simulink model "Velocity"  (R2023b)
settings: Solver=VariableStepAuto  StartTime=0.0  StopTime=10.0  RelTol=1e-3
undefined symbols (not defined in the file): g
libraries: simulink x3, eeGeneralControl x1
settings Model: Creator=Saif Mohamed  LastModifiedBy=saifg

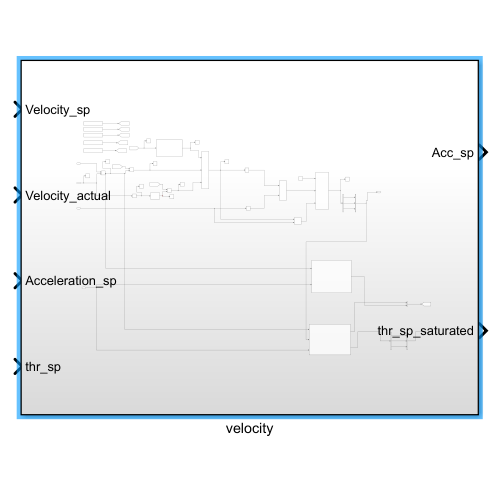
[thumbnail: Simulink's stored preview of the top-level diagram]
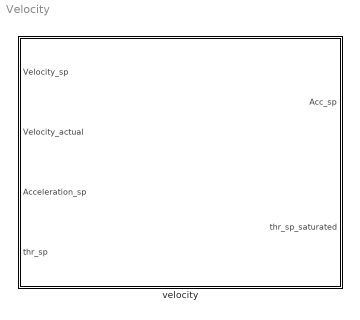
== system Velocity ==
  velocity : Subsystem

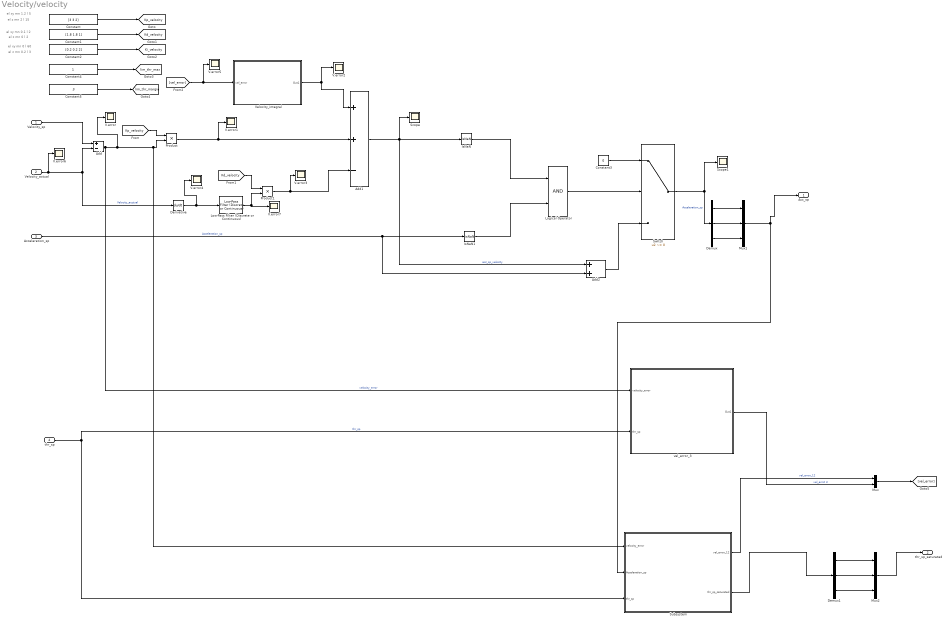
== system Velocity/velocity ==
  note: el z mn 0.2 l 3
  note: el xy mn 0 l 60
  note: el xy mn 0.1 l 2
  note: el z mn 0 l 2
  note: el xy mn 1.2 l 5
  note: el z mn 2 l 15
  Velocity_sp : Inport
  Velocity_actual : Inport  Port=2
  Acceleration_sp : Inport  Port=3
  thr_sp : Inport  Port=4
  Add : Sum  Inputs=+-
  Add1 : Sum  Inputs=++-
  Add2 : Sum
  Constant : Constant  Value=[3 3 2]
  Constant1 : Constant  Value=[1.8 1.8 1]
  Constant2 : Constant  Value=[0.2 0.2 2]
  Constant3 : Constant  Value=0
  Constant4 : Constant
  Constant5 : Constant  Value=.3
  Demux : Demux  Outputs=3
  Demux1 : Demux  Outputs=3
  Derivative : Derivative
  IsNaN : RelationalOperator  Operator=isNaN  OutDataTypeStr=boolean  RndMeth=Simplest  InputSameDT=off
  IsNaN1 : RelationalOperator  Operator=isNaN  OutDataTypeStr=boolean  RndMeth=Simplest  InputSameDT=off
  Logical Operator : Logic  AllPortsSameDT=off  OutDataTypeStr=boolean
  Low-Pass Filter (Discrete or Continuous) : eeGeneralControl/Low-Pass Filter (Discrete or Continuous)  K=1  T=1  B=inf  A=-inf  init_option=Inherited from block input  x0=0  Ts=-1
  Mux : Mux  Inputs=2
  Mux1 : Mux  Inputs=3
  Mux2 : Mux  Inputs=3
  Product : Product
  Product1 : Product
  Scope : Scope
  Scope1 : Scope
  Subsystem : Subsystem
  Switch : Switch  Criteria=u2 ~= 0  SaturateOnIntegerOverflow=off  InputSameDT=off
  V.error{,1..7} (8 alike) : Scope
  Velocity_integral : Subsystem
  vel_error_3 : Subsystem
  Acc_sp : Outport
  thr_sp_saturated : Outport  Port=2
  tag scope: Kd_velocity=global, Ki_velocity=global, Kp_velocity=global, lim_thr_margin=global, lim_thr_max=global
  wires:
  Velocity_sp/1 -> Add/1
  Velocity_actual/1 -> V.error6/1, Derivative/1, Add/2  "Velocity_acctual"
  Add/1 -> vel_error_3/1(velocity_error), V.error/1, Subsystem/1(velocity_error), Product/2  "velocity_error"
  Constant/1 -> [Kp_velocity]
  [Kp_velocity] -> Product/1
  Derivative/1 -> V.error4/1, Low-Pass Filter (Discrete or Continuous)/1
  Constant1/1 -> [Kd_velocity]
  Low-Pass Filter (Discrete or Continuous)/1 -> V.error7/1, Product1/2
  [Kd_velocity] -> Product1/1
  Constant2/1 -> [Ki_velocity]
  Add1/1 -> Scope/1, IsNaN/1, Add2/1  "acc_sp_velocity"
  Acceleration_sp/1 -> Add2/2, IsNaN1/1  "Acceleration_sp"
  IsNaN1/1 -> Logical Operator/2
  IsNaN/1 -> Logical Operator/1
  Logical Operator/1 -> Switch/2
  Add2/1 -> Switch/3
  Constant3/1 -> Switch/1
  Switch/1 -> Scope1/1, Demux/1  "Acceleration_sp"
  Constant4/1 -> [lim_thr_max]
  thr_sp/1 -> Subsystem/3(thr_sp), vel_error_3/2(thr_sp)  "thr_sp"
  vel_error_3/1(Out1) -> Mux/2  "vel_errot 3"
  Constant5/1 -> [lim_thr_margin]
  Subsystem/1(vel_error_12) -> Mux/1  "vel_error_12"
  Mux/1 -> [vel_error]
  Demux/3 -> Mux1/3
  Demux/2 -> Mux1/2
  Demux/1 -> Mux1/1
  Demux1/1 -> Mux2/1
  Demux1/2 -> Mux2/2
  Subsystem/2(thr_sp_satureted) -> Demux1/1
  Mux2/1 -> thr_sp_saturated/1
  Demux1/3 -> Mux2/3
  Product/1 -> Add1/2, V.error1/1
  Velocity_integral/1(Out1) -> Add1/1, V.error2/1
  Product1/1 -> Add1/3, V.error3/1
  Mux1/1 -> Subsystem/2(Acceleration_sp), Acc_sp/1
  [vel_error] -> Velocity_integral/1(vel_error), V.error5/1

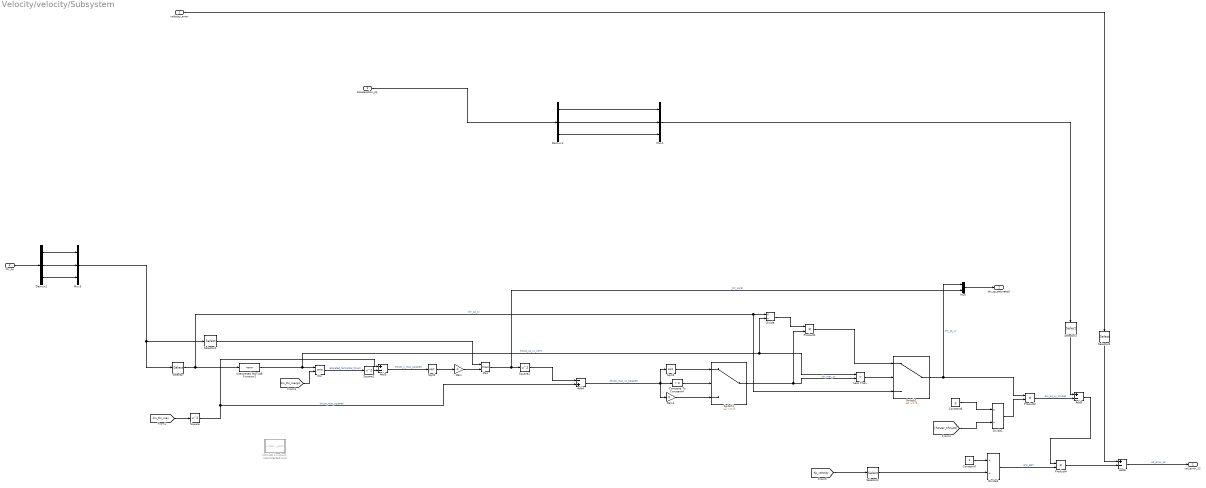
== system Velocity/velocity/Subsystem ==
  velocity_error : Inport
  Acceleration_sp : Inport  Port=2
  thr_sp : Inport  Port=3
  Add3 : Sum  Inputs=+-
  Add4 : Sum  Inputs=-+
  Add5 : Sum  Inputs=+-
  Add6 : Sum  Inputs=+-
  Compare To Constant4 : simulink/Logic and Bit Operations/Compare To Constant  relop=>  const=0  OutDataTypeStr=boolean
  Constant6 : Constant  Value=g
  Constant7 : Constant  Value=2
  Demux1 : Demux  Outputs=3
  Demux2 : Demux  Outputs=3
  Divide : Product  Inputs=*/
  Divide1 : Product  Inputs=*/
  Divide2 : Product  Inputs=*/
  Gain : Gain  Gain=-1
  Gain1 : Gain  Gain=0
  Interpreted MATLAB Function1 : MATLABFcn  MATLABFcn=norm
  Less Than : RelationalOperator  Operator=>  OutDataTypeStr=boolean  RndMeth=Simplest  InputSameDT=off
  MATLAB Function1 : MATLAB Function  Commented=on  TreatAsAtomicUnit=on
  Max : MinMax  Function=max  Inputs=2
  Min : MinMax  Inputs=2
  Mux : Mux  Inputs=2
  Mux1 : Mux  Inputs=3
  Mux3 : Mux  Inputs=3
  Product2 : Product
  Product3 : Product
  Product4 : Product
  Selector : Selector  InputPortWidth=3  IndexOptions=Index vector (dialog)  Indices=[1 2]  OutputSizes=1
  Selector1 : Selector  InputPortWidth=3  IndexOptions=Index vector (dialog)  Indices=[3]  OutputSizes=1
  Selector2 : Selector  InputPortWidth=3  IndexOptions=Index vector (dialog)  Indices=[1]  OutputSizes=1
  Selector3 : Selector  InputPortWidth=3  IndexOptions=Index vector (dialog)  Indices=[1 2]  OutputSizes=1
  Selector4 : Selector  InputPortWidth=3  IndexOptions=Index vector (dialog)  Indices=[1 2]  OutputSizes=1
  Sqrt1 : Sqrt
  Sqrt3 : Sqrt
  Square : Math  Operator=square
  Square1 : Math  Operator=square
  Square2 : Math  Operator=square
  Switch1 : Switch  Criteria=u2 ~= 0  Threshold=~0  SaturateOnIntegerOverflow=off  InputSameDT=off
  Switch2 : Switch  Criteria=u2 ~= 0  Threshold=~0  SaturateOnIntegerOverflow=off  InputSameDT=off
  vel_error_12 : Outport
  thr_sp_satureted : Outport  Port=2
  wires:
  Square/1 -> Add4/2, Add3/1  "thrust_max_squared"
  Divide2/1 -> Product4/2  "arw_gain"
  Selector/1 -> Interpreted MATLAB Function1/1, Switch2/3, Divide/1  "thr_sp_xy"
  Add5/1 -> Product4/1
  Max/1 -> Square2/1, Mux/2  "_thr_sp(3)"
  Product4/1 -> Add6/2
  Divide/1 -> Product2/1
  Compare To Constant4/1 -> Switch1/2
  Sqrt3/1 -> Switch1/1
  Selector4/1 -> Add6/1
  Switch2/1 -> Mux/1, Product3/1  "thr_sp_xy"
  Interpreted MATLAB Function1/1 -> Divide/2, Less Than/1, Min/1  "thrust_sp_xy_norm"
  Add4/1 -> Gain1/1, Sqrt3/1, Compare To Constant4/1  "thrust_max_xy_squared"
  Selector1/1 -> Max/1
  Sqrt1/1 -> Gain/1
  Selector2/1 -> Divide2/2
  Switch1/1 -> Product2/2, Less Than/2  "thr_max_xy"
  [lim_thr_max] -> Square/1
  [hover_thrust] -> Divide1/2
  Add3/1 -> Sqrt1/1  "thrust_z_max_squared"
  Selector3/1 -> Add5/1
  Gain/1 -> Max/2
  [lim_thr_margin] -> Min/2
  Product2/1 -> Switch2/1
  Product3/1 -> Add5/2  "acc_sp_xy_limited"
  [Kp_velocity] -> Selector2/1
  Square2/1 -> Add4/1
  Less Than/1 -> Switch2/2
  Constant7/1 -> Divide2/1
  Min/1 -> Square1/1  "allocated_horizontal_thrust"
  Divide1/1 -> Product3/2
  Add6/1 -> vel_error_12/1  "vel_error_12"
  velocity_error/1 -> Selector4/1
  Square1/1 -> Add3/2
  Constant6/1 -> Divide1/1
  Gain1/1 -> Switch1/3
  Mux/1 -> thr_sp_satureted/1
  Demux2/1 -> Mux3/1
  Demux2/2 -> Mux3/2
  Mux3/1 -> Selector/1, Selector1/1
  thr_sp/1 -> Demux2/1
  Demux2/3 -> Mux3/3
  Mux1/1 -> Selector3/1
  Acceleration_sp/1 -> Demux1/1
  Demux1/3 -> Mux1/3
  Demux1/2 -> Mux1/2
  Demux1/1 -> Mux1/1

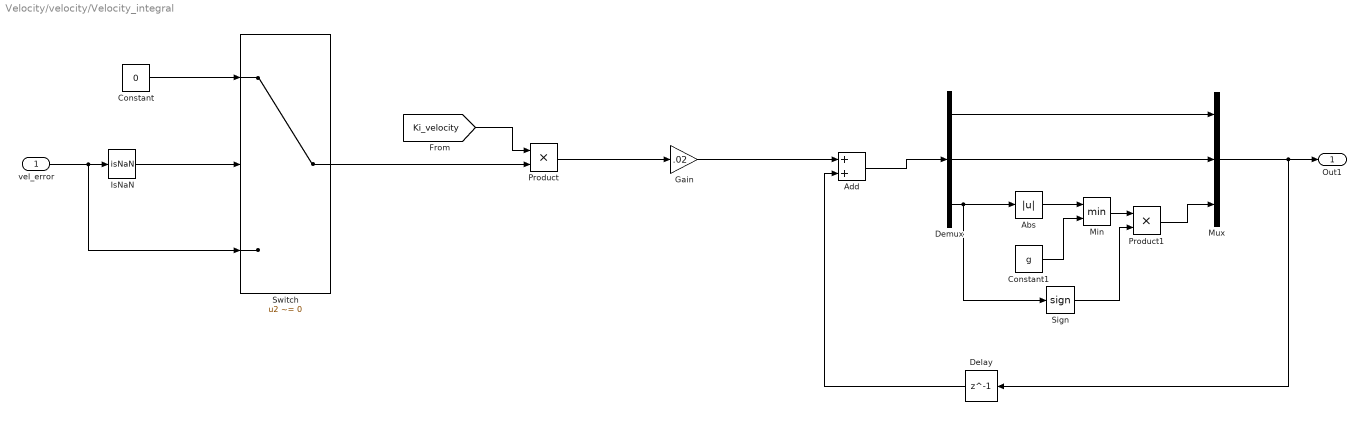
== system Velocity/velocity/Velocity_integral ==
  vel_error : Inport
  Abs : Abs  SaturateOnIntegerOverflow=off
  Add : Sum
  Constant : Constant  Value=0
  Constant1 : Constant  Value=g
  Delay : Delay  DelayLength=1
  Demux : Demux  Outputs=3
  Gain : Gain  Gain=.02
  IsNaN : RelationalOperator  Operator=isNaN  OutDataTypeStr=boolean  RndMeth=Simplest  InputSameDT=off
  Min : MinMax  Inputs=2
  Mux : Mux  Inputs=3
  Product : Product
  Product1 : Product
  Sign : Signum
  Switch : Switch  Criteria=u2 ~= 0  SaturateOnIntegerOverflow=off  InputSameDT=off
  Out1 : Outport
  wires:
  vel_error/1 -> Switch/3, IsNaN/1
  IsNaN/1 -> Switch/2
  Constant/1 -> Switch/1
  [Ki_velocity] -> Product/1
  Switch/1 -> Product/2
  Delay/1 -> Add/2
  Min/1 -> Product1/1
  Constant1/1 -> Min/2
  Product1/1 -> Mux/3
  Abs/1 -> Min/1
  Gain/1 -> Add/1
  Demux/3 -> Sign/1, Abs/1
  Sign/1 -> Product1/2
  Add/1 -> Demux/1
  Product/1 -> Gain/1
  Demux/2 -> Mux/2
  Demux/1 -> Mux/1
  Mux/1 -> Out1/1, Delay/1

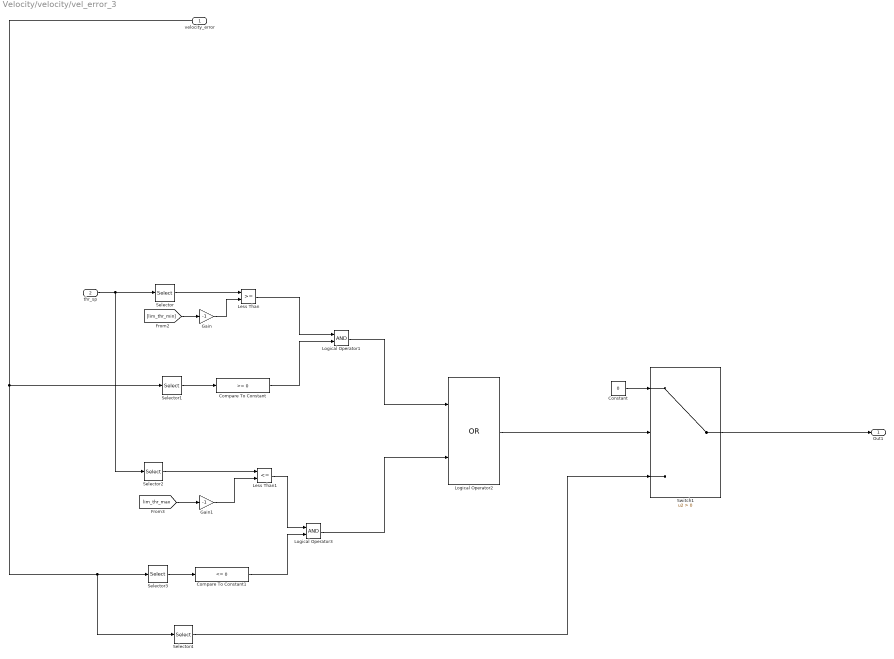
== system Velocity/velocity/vel_error_3 ==
  velocity_error : Inport
  thr_sp : Inport  Port=2
  Compare To Constant : simulink/Logic and Bit Operations/Compare To Constant  relop=>=  const=0  OutDataTypeStr=boolean
  Compare To Constant1 : simulink/Logic and Bit Operations/Compare To Constant  relop=<=  const=0  OutDataTypeStr=boolean
  Constant : Constant  Value=0
  Gain : Gain  Gain=-1
  Gain1 : Gain  Gain=-1
  Less Than : RelationalOperator  OutDataTypeStr=boolean  RndMeth=Simplest  InputSameDT=off
  Less Than1 : RelationalOperator  Operator=<=  OutDataTypeStr=boolean  RndMeth=Simplest  InputSameDT=off
  Logical Operator1 : Logic  AllPortsSameDT=off  OutDataTypeStr=boolean
  Logical Operator2 : Logic  Operator=OR  AllPortsSameDT=off  OutDataTypeStr=boolean
  Logical Operator3 : Logic  AllPortsSameDT=off  OutDataTypeStr=boolean
  Selector{,1..4} (5 alike) : Selector  InputPortWidth=3  IndexOptions=Index vector (dialog)  Indices=[3]  OutputSizes=1
  Switch1 : Switch  Criteria=u2 > Threshold  SaturateOnIntegerOverflow=off  InputSameDT=off
  Out1 : Outport
  wires:
  Less Than1/1 -> Logical Operator3/1
  velocity_error/1 -> Selector4/1, Selector3/1, Selector1/1
  Compare To Constant/1 -> Logical Operator1/2
  thr_sp/1 -> Selector2/1, Selector/1
  [lim_thr_min] -> Gain/1
  [lim_thr_max] -> Gain1/1
  Selector/1 -> Less Than/1
  Logical Operator1/1 -> Logical Operator2/1
  Compare To Constant1/1 -> Logical Operator3/2
  Selector1/1 -> Compare To Constant/1
  Selector2/1 -> Less Than1/1
  Gain/1 -> Less Than/2
  Selector3/1 -> Compare To Constant1/1
  Logical Operator2/1 -> Switch1/2
  Less Than/1 -> Logical Operator1/1
  Gain1/1 -> Less Than1/2
  Logical Operator3/1 -> Logical Operator2/2
  Switch1/1 -> Out1/1
  Selector4/1 -> Switch1/3
  Constant/1 -> Switch1/1

== matlab function Velocity/velocity/Subsystem/MATLAB Function1 ==
  data: u input; thrust_sp_xy_norm output
function thrust_sp_xy_norm = fcn(u)
thrust_sp_xy_norm=norm(u);
end
